simulink model "Papersim_mitigation"  (R2025a)
settings: Solver=ode23tb  StartTime=0.0  StopTime=0.3  MaxStep=1e-5  RelTol=1e-3
undefined symbols (not defined in the file): D11, Delta
libraries: spsRMSLib x5, spsACCurrentSourceLib x3, spsIdealSwitchLib x3, spsVoltageMeasurementLib x2, spsCurrentMeasurementLib x1, spsGroundLib x1, spsThreePhasePISectionLineLib x1, spsThreePhaseParallelRLCLoadLib x1, spsThreePhaseVIMeasurementLib x1, spsThreePhaseSourceLib x1, spsThreePhaseTransformerTwoWindingsLib x1, sps_lib x1
settings Model: Creator=ADMIN  LastModifiedBy=ADMIN

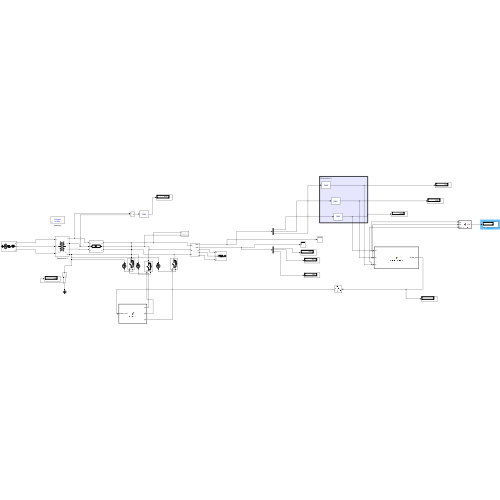
[thumbnail: Simulink's stored preview of the top-level diagram]
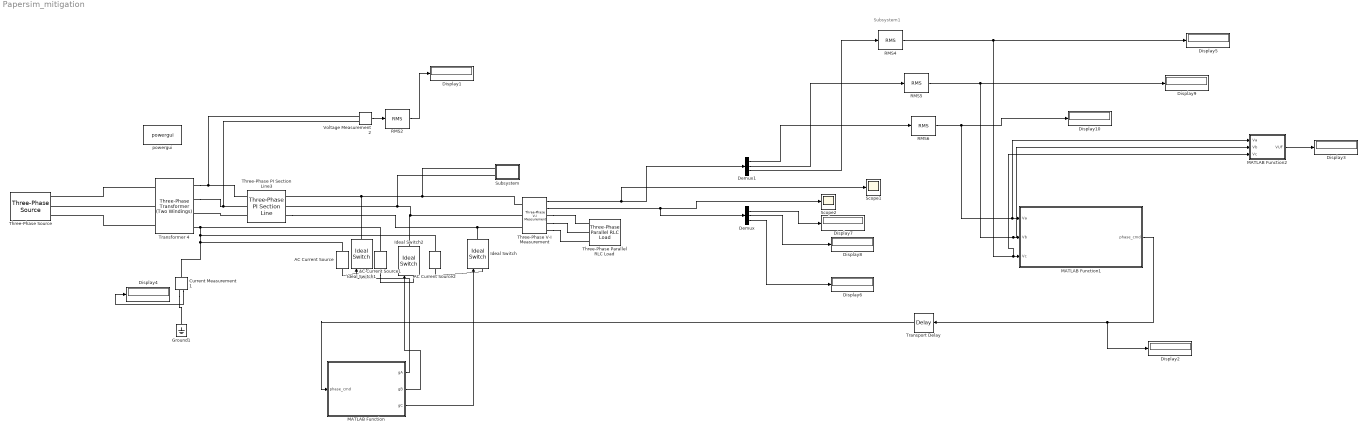
== system Papersim_mitigation ==
  note: Subsystem1
  AC Current Source : spsACCurrentSourceLib/AC Current Source  Amplitude=236  Phase=0  Frequency=50  SampleTime=0  Measurements=None
      settings: LibrarySourceBlock=sps_lib/Sources/AC Current Source
  AC Current Source1 : spsACCurrentSourceLib/AC Current Source  Amplitude=236  Phase=-120  Frequency=50  SampleTime=0  Measurements=None
      settings: LibrarySourceBlock=sps_lib/Sources/AC Current Source
  AC Current Source2 : spsACCurrentSourceLib/AC Current Source  Amplitude=236  Phase=120  Frequency=50  SampleTime=0  Measurements=None
      settings: LibrarySourceBlock=sps_lib/Sources/AC Current Source
  Current Measurement1 : spsCurrentMeasurementLib/Current Measurement  PhasorSimulation=off  OutputType=Complex  PSBequivalent=0
  Demux : Demux  Outputs=3
  Demux1 : Demux  Outputs=3
  Display{1..10} (10 alike) : Display
  Ground1 : spsGroundLib/Ground  LConnTagsString=a
  Ideal Switch : spsIdealSwitchLib/Ideal Switch  Ron=0.001  Lon=0  IC=0  Rs=1e5  Cs=inf  Measurements=off
  Ideal Switch1 : spsIdealSwitchLib/Ideal Switch  Ron=0.001  Lon=0  IC=0  Rs=1e5  Cs=inf  Measurements=off
  Ideal Switch2 : spsIdealSwitchLib/Ideal Switch  Ron=0.001  Lon=0  IC=0  Rs=1e5  Cs=inf  Measurements=off
  MATLAB Function : MATLAB Function  TreatAsAtomicUnit=on
  MATLAB Function1 : MATLAB Function  TreatAsAtomicUnit=on
  MATLAB Function2 : MATLAB Function  TreatAsAtomicUnit=on
  RMS{2,4..6} (4 alike) : spsRMSLib/RMS  TrueRMS=on  Freq=50  RMSInit=120  Ts=0
  Scope1 : Scope
      settings: ActiveDisplayYMinimum=-502.36255036020566  ActiveDisplayYMaximum=404.46999737979149
  Scope2 : Scope
      settings: ActiveDisplayYMinimum=-664.9159508382179  ActiveDisplayYMaximum=991.3973704981795  DataLoggingVariableName=ScopeData2
  Subsystem : Subsystem
  Three-Phase PI Section Line3 : spsThreePhasePISectionLineLib/Three-Phase PI Section Line  LConnTagsString=a|b|c  RConnTagsString=A|B|C  Length=1.2  Frequency=50  Resistances=[0.01377 0.04131 ]  Inductances=[31.83e-6 95.49e-6]  Capacitances=[250e-9 80e-9]
  Three-Phase Parallel RLC Load : spsThreePhaseParallelRLCLoadLib/Three-Phase Parallel RLC Load  LConnTagsString=A|B|C  Configuration=Y (grounded)  NominalVoltage=415  Vabc=[239.6 239.6 239.6]  Vabcp=[1e3 1e3 1e3]  NominalFrequency=50  UnbalancedPower=on  ActivePower=6000  InductivePower=2500  CapacitivePower=0  Pabc="[32.1e3 52.5e3  72.5e3]"  QLabc=[0 0 0]  QCabc=[0 0 0 ]  Pabcp=[10e3 9e3 11e3]  QLabcp=[100 90 110]  QCabcp=[100 90 110]  Measurements=None  LoadType=constant PQ
  Three-Phase V-I Measurement : spsThreePhaseVIMeasurementLib/Three-Phase V-I Measurement  VoltageMeasurement=phase-to-ground  SetLabelV=off  LabelV=Vabc  Vpu=off  VpuLL=off  CurrentMeasurement=yes  SetLabelI=off  LabelI=Iabc  Ipu=off  Pbase=100e6  Vbase=500e3  OutputType=Complex  PhasorSimulation=off  PSBequivalent=0
  Three-Phase Source : spsThreePhaseSourceLib/Three-Phase Source  InternalConnection=Yg  VoltagePhases=off  Voltage=11000  PhaseAngle=0  Voltage_phases=[25e3 25e3 25e3]/sqrt(3)  PhaseAngles_phases=[0 -120 +120]  Frequency=50  NonIdealSource=on  SpecifyImpedance=on  Resistance=0.01  Inductance=0.1  ShortCircuitLevel=10e6  BaseVoltage=11e3  XRratio=7  BusType=swing  Pref=10e3  Qref=0  Prefabc=[10e3, 10e3, 10e3]  Qrefabc=[0, 0, 0]  Qmin=-inf  Qmax=inf
  Transformer 4 : spsThreePhaseTransformerTwoWindingsLib/Three-Phase Transformer (Two Windings)  Winding1Connection=Delta (D11)  Winding2Connection=Yn  CoreType=Three single-phase transformers  SetSaturation=off  Hysteresis=off  DataFile='hysteresis'  SetInitialFlux=off  Measurements=None  UNITS=pu  NominalPower=[ 200e3 , 50 ]  Winding1=[11000 0.01 0.08]  Winding2=[415 0.01 0.08]  Rm=500  Lm=500  L0=0.39999  Saturation=[0 0;0.003 1.2;1.25 1.52]  InitialFluxes=[0.8 -0.8 0.7]  BreakLoop=off  DiscreteSolver=Trapezoidal iterative  DataType=off  TransfoNumber=1
  Transport Delay : TransportDelay  DelayTime=0.1
  Voltage Measurement2 : spsVoltageMeasurementLib/Voltage Measurement  PhasorSimulation=off  OutputType=Complex  PSBequivalent=0
  powergui : sps_lib/powergui  Priority=1  SimulationMode=Discrete  SampleTime=5e-6  frequency=50  Iterations=50  frequencyindice=50  Pbase=100e6  ErrMax=1e-4  UnitsV=kV  UnitsW=MW  buscounter=0  FunctionMessages=off  echomessages=off  EnableUseOfTLC=off  CurrentSourceSwitches=off  DisableSnubberDevices=off  DisableRonSwitches=off  DisableVfSwitches=off  DisplayEquations=off  AutomaticDiscreteSolvers=off  SolverType=Tustin/Backward Euler (TBE)  Interpol=off  ExternalGateDelay=off  methode=off  Ts=100  x0status=blocks  SPID=on  SwTol=0  HookPort=off  NonlinearTolerance=1e-4  nMaxIteration=100  ContinueOnMaxIteration=off  RestoreLinks=warning  ResistiveCurrentMeasurement=off  Frange=[0:2:500]  Ylog=off  Xlog=on  ShowGrid=off  save=off  variable=ZData  structure=0  ZoomFFT=off  StartTime=0.0  cycles=1  DisplayStyle=1  fundamental=60  FreqAxis=off  MaxFrequency=1000  frequencyindicesteady=1  RmsSteady=1  display=off
  wires:
  Voltage Measurement2/1 -> RMS2/1
  RMS2/1 -> Display1/1
  Three-Phase V-I Measurement/1 -> Demux1/1, Scope1/1
  Three-Phase V-I Measurement/2 -> Scope2/1, Demux/1
  Demux/1 -> Display7/1
  Demux/2 -> Display8/1
  Demux/3 -> Display6/1
  Current Measurement1/1 -> Display4/1
  Demux1/2 -> RMS5/1
  Demux1/3 -> RMS4/1
  Demux1/1 -> RMS6/1
  RMS4/1 -> MATLAB Function2/3(Vc), MATLAB Function1/3(Vc), Display5/1
  RMS5/1 -> MATLAB Function2/2(Vb), MATLAB Function1/2(Vb), Display9/1
  RMS6/1 -> MATLAB Function2/1(Va), MATLAB Function1/1(Va), Display10/1
  MATLAB Function1/1(phase_cmd) -> Display2/1, Transport Delay/1
  MATLAB Function/1(gA) -> Ideal Switch1/1
  MATLAB Function/2(gB) -> Ideal Switch2/1
  MATLAB Function/3(gC) -> Ideal Switch/1
  Transport Delay/1 -> MATLAB Function/1(phase_cmd)
  MATLAB Function2/1(VUF) -> Display3/1
  connections:
  Transformer 4/LConn2 -- Three-Phase Source/RConn2
  Transformer 4/LConn1 -- Three-Phase Source/RConn1
  Transformer 4/LConn3 -- Three-Phase Source/RConn3
  Transformer 4/RConn1 -- Voltage Measurement2/LConn1 -- Three-Phase PI Section Line3/LConn1
  Transformer 4/RConn2 -- Three-Phase PI Section Line3/LConn2 -- Voltage Measurement2/LConn2
  Three-Phase PI Section Line3/LConn3 -- Transformer 4/RConn3
  Three-Phase V-I Measurement/RConn1 -- Three-Phase Parallel RLC Load/LConn1
  Three-Phase V-I Measurement/RConn2 -- Three-Phase Parallel RLC Load/LConn2
  Three-Phase V-I Measurement/RConn3 -- Three-Phase Parallel RLC Load/LConn3
  Three-Phase PI Section Line3/RConn3 -- Ideal Switch/RConn1 -- Three-Phase V-I Measurement/LConn3
  Three-Phase V-I Measurement/LConn1 -- Subsystem/LConn1 -- Ideal Switch1/RConn1 -- Three-Phase PI Section Line3/RConn1
  Three-Phase V-I Measurement/LConn2 -- Ideal Switch2/RConn1 -- Three-Phase PI Section Line3/RConn2 -- Subsystem/LConn2
  Current Measurement1/RConn1 -- Ground1/LConn1
  Transformer 4/RConn4 -- AC Current Source1/RConn1 -- AC Current Source2/RConn1 -- AC Current Source/RConn1 -- Current Measurement1/LConn1
  AC Current Source2/LConn1 -- Ideal Switch/LConn1
  AC Current Source1/LConn1 -- Ideal Switch2/LConn1
  AC Current Source/LConn1 -- Ideal Switch1/LConn1

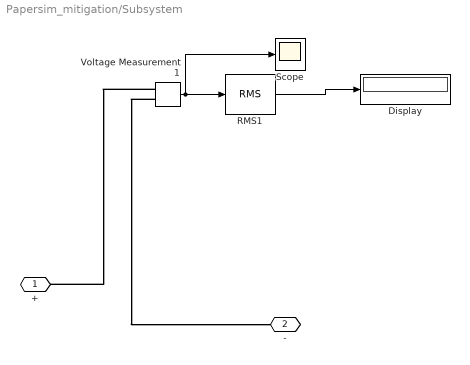
== system Papersim_mitigation/Subsystem ==
  Display : Display
  RMS1 : spsRMSLib/RMS  TrueRMS=on  Freq=50  RMSInit=120  Ts=0
  Scope : Scope
      settings: ActiveDisplayYMinimum=-999.7877288425824  ActiveDisplayYMaximum=1157.6057893237362
  Voltage Measurement1 : spsVoltageMeasurementLib/Voltage Measurement  PhasorSimulation=off  OutputType=Complex  PSBequivalent=0
  + : PMIOPort  Side=Left
  - : PMIOPort  Port=2  Side=Left
  wires:
  Voltage Measurement1/1 -> Scope/1, RMS1/1
  RMS1/1 -> Display/1
  connections:
  Voltage Measurement1/LConn1 -- +/RConn1
  Voltage Measurement1/LConn2 -- -/RConn1

== matlab function Papersim_mitigation/MATLAB Function1 ==
  settings: updateMethod=DISCRETE
  data: Va input; Vb input; phase_cmd output; Vc input
function phase_cmd = phase_controller(Va, Vb, Vc)

persistent prev_phase;

if isempty(prev_phase)
    prev_phase = 1;   % Start with Phase A
end

% --- VUF Calculation ---
Vavg = (Va + Vb + Vc)/3;
dev = [abs(Va - Vavg), abs(Vb - Vavg), abs(Vc - Vavg)];
VUF = (max(dev) / Vavg) * 100;

% --- Hysteresis ---
upper = 3;   % switching threshold
lower = 2;   % deadband

if VUF < lower
    phase_cmd = prev_phase;
    return;
end

if VUF > upper
    % Find underloaded phase (LOWEST voltage)
    [~, underloaded] = min([Va, Vb, Vc]);

    phase_cmd = underloaded;

    % update memory
    prev_phase = phase_cmd;
else
    phase_cmd = prev_phase;
end

end

== matlab function Papersim_mitigation/MATLAB Function ==
  data: phase_cmd input; gA output; gB output; gC output
function [gA, gB, gC] = decoder(phase_cmd)
% Convert phase command to individual switch gate signals
gA = double(phase_cmd == 1);  % 1 if connect to Phase A
gB = double(phase_cmd == 2);  % 1 if connect to Phase B  
gC = double(phase_cmd == 3);  % 1 if connect to Phase C
end

== matlab function Papersim_mitigation/MATLAB Function2 ==
  data: Va input; VUF output; Vb input; Vc input
function VUF = calc_VUF(Va, Vb, Vc)

Vavg = (Va + Vb + Vc)/3;

devA = abs(Va - Vavg);
devB = abs(Vb - Vavg);
devC = abs(Vc - Vavg);

max_dev = max([devA, devB, devC]);

VUF = (max_dev / Vavg) * 100;

end
